simulink model "model2lab2"  (Simulink 7.9)
settings: Solver=ode4  StartTime=0.0  StopTime=100  FixedStep=0.01  RelTol=1e-3
settings Model: Creator=gglowacki  LastModifiedBy=aziemba

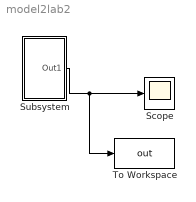
== system model2lab2 ==
  Scope : Scope
  Subsystem : Subsystem  mask{g=10, l=3, k=1, m=10, fi0=90, to=0}
      mask prompts: g "grawitacja"; l "dlugosc_wahadla"; k "wsp.tlumienia"; m "masa_wahadla"; fi0 "kat_odchylenia"; to "czas_symulacji"
  To Workspace : ToWorkspace  VariableName=out  SampleTime=-1  SaveFormat=Timeseries
  wires:
  Subsystem/1(Out1) -> Scope/1, To Workspace/1

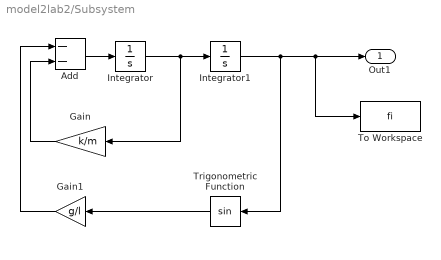
== system model2lab2/Subsystem ==
  Add : Sum  Inputs=--
  Gain : Gain  Gain=k/m
  Gain1 : Gain  Gain=g/l
  Integrator : Integrator
  Integrator1 : Integrator  InitialCondition=(fi0*pi)/180
  To Workspace : ToWorkspace  VariableName=fi  SampleTime=-1  SaveFormat=Timeseries
  Trigonometric Function : Trigonometry
  Out1 : Outport
  wires:
  Integrator/1 -> Integrator1/1, Gain/1
  Add/1 -> Integrator/1
  Gain/1 -> Add/2
  Integrator1/1 -> Trigonometric Function/1, Out1/1, To Workspace/1
  Trigonometric Function/1 -> Gain1/1
  Gain1/1 -> Add/1
